simulink model "simple_switch_model"  (R2023b)
settings: Solver=VariableStepAuto  StartTime=0.0  StopTime=10.0  RelTol=1e-3
settings Model: Creator=39216  LastModifiedBy=39216

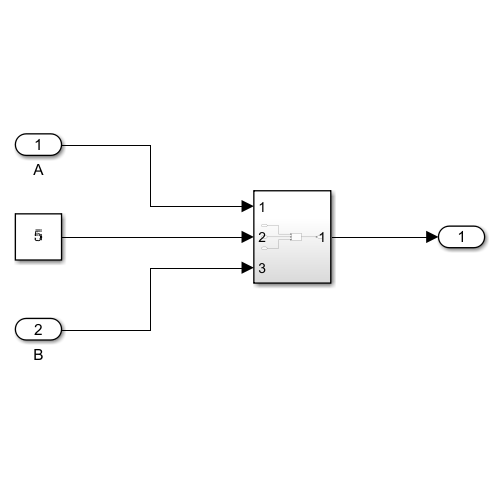
[thumbnail: Simulink's stored preview of the top-level diagram]
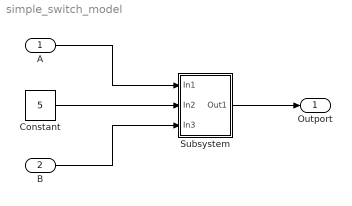
== system simple_switch_model ==
  A : Inport
  B : Inport  Port=2
  Constant : Constant  Value=5
  Subsystem : Subsystem
  Outport : Outport
  wires:
  A/1 -> Subsystem/1(In1)
  Constant/1 -> Subsystem/2(In2)
  B/1 -> Subsystem/3(In3)
  Subsystem/1(Out1) -> Outport/1

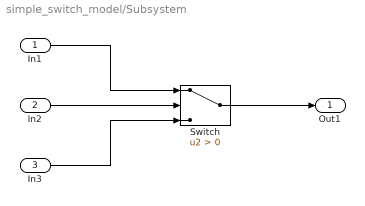
== system simple_switch_model/Subsystem ==
  In1 : Inport
  In2 : Inport  Port=2
  In3 : Inport  Port=3
  Switch : Switch  Criteria=u2 > Threshold  SaturateOnIntegerOverflow=off  InputSameDT=off
  Out1 : Outport
  wires:
  In2/1 -> Switch/2
  Switch/1 -> Out1/1
  In3/1 -> Switch/3
  In1/1 -> Switch/1
